simulink model "exc2_e"  (R2015a)
settings: Solver=ode45  StartTime=0.0  StopTime=2  RelTol=1e-3
values from neighbouring files (symbols this model uses):
  A5 = [0 1 0 0;20.9 0 0 0;0 0 0 1;-0.8 0 0 0]    [ask2_A.m]
  B = [0;-1;0;0.5]    [ask2_A.m]
  C = [1 0 0 0;0 0 1 0]    [ask2_A.m]
  initial = [-0.2;-0.06;0.01;0.3]    [ask2_A.m]
  K1 = (ad-a0)*T    [ask2_A.m]
settings Model: Creator=Γιώργος  LastModifiedBy=Γιώργος
settings DataIOCC: FinalStateName=xFinal5  SaveFinalState=on  SaveState=on  StateSaveName=xout5  TimeSaveName=tout5  OutputSaveName=yout5

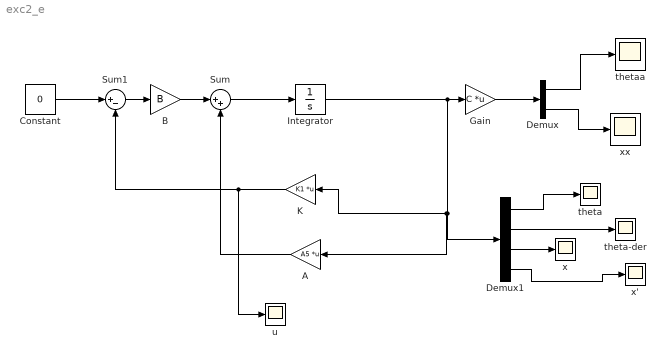
== system exc2_e ==
  A : Gain  Gain=A5  Multiplication=Matrix(K*u)
  B : Gain  Gain=B
  Constant : Constant  Value=0
  Demux : Demux  Outputs=2
  Demux1 : Demux
  Gain : Gain  Gain=C  Multiplication=Matrix(K*u) (u vector)
  Integrator : Integrator  InitialCondition=initial
  K : Gain  Gain=K1  Multiplication=Matrix(K*u)
  Sum : Sum  Inputs=|++
  Sum1 : Sum  Inputs=|+-
  theta : Scope
      settings: SaveName=ScopeData2
  theta-der : Scope
      settings: SaveName=ScopeData3
  thetaa : Scope
  u : Scope
      settings: SaveName=ScopeData6
  x : Scope
      settings: SaveName=ScopeData4
  "x' " : Scope
      settings: SaveName=ScopeData5
  xx : Scope
  wires:
  Gain/1 -> Demux/1
  Demux/1 -> thetaa/1
  Demux/2 -> xx/1
  A/1 -> Sum/2
  Sum/1 -> Integrator/1
  K/1 -> Sum1/2, u/1
  Constant/1 -> Sum1/1
  Sum1/1 -> B/1
  B/1 -> Sum/1
  Integrator/1 -> Demux1/1, A/1, K/1, Gain/1
  Demux1/1 -> theta/1
  Demux1/2 -> theta-der/1
  Demux1/3 -> x/1
  Demux1/4 -> "x' "/1
